simulink model "simulink_q9"  (R2020a)
settings: Solver=VariableStepAuto  StartTime=0.0  StopTime=50  RelTol=1e-3
libraries: simulink x1
settings Model: Creator=debora  LastModifiedBy=debora

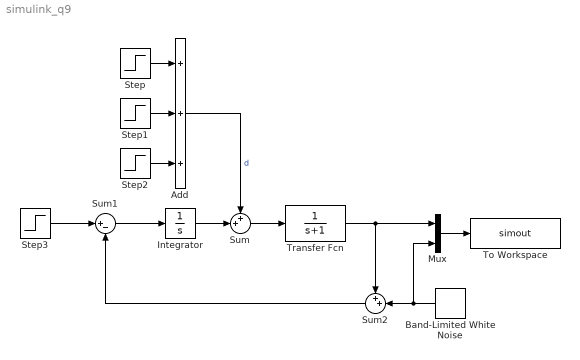
== system simulink_q9 ==
  Add : Sum  Inputs=3
  Band-Limited White Noise : simulink/Sources/Band-Limited White Noise  Cov=[0.01]  Ts=0.1  seed=[23341]
  Integrator : Integrator
  Mux : Mux  Inputs=2
  Step : Step  Time=0  After=-1  SampleTime=0
  Step1 : Step  Time=6  After=3  SampleTime=0
  Step2 : Step  Time=15  After=-1  SampleTime=0
  Step3 : Step  Time=0  SampleTime=0
  Sum : Sum  Inputs=++|
  Sum1 : Sum  Inputs=|+-
  Sum2 : Sum  Inputs=++|
  To Workspace : ToWorkspace  VariableName=simout  SaveFormat=Timeseries  SampleTime=-1
  Transfer Fcn : TransferFcn  Denominator=[1 1]
  wires:
  Integrator/1 -> Sum/2
  Step/1 -> Add/1
  Step1/1 -> Add/2
  Step2/1 -> Add/3
  Add/1 -> Sum/1  "d"
  Sum/1 -> Transfer Fcn/1
  Sum1/1 -> Integrator/1
  Step3/1 -> Sum1/1
  Transfer Fcn/1 -> Mux/1, Sum2/1
  Sum2/1 -> Sum1/2
  Band-Limited White Noise/1 -> Mux/2, Sum2/2
  Mux/1 -> To Workspace/1
